simulink model "uGrid_1PH_hd_ATD3"  (R2018a)
settings: Solver=ode45  StartTime=0.0  StopTime=1.5  FixedStep=1e-6  MaxStep=1e-4  RelTol=1e-3
PreLoadFcn:
  | SimulinkInit
InitFcn:
  | SimulinkInit
StopFcn:
  | EndingScript
values from neighbouring files (symbols this model uses):
  Ad = sysd.A    [SimulinkInit.m]
  b = 4.91    [SimulinkInit.m]    (also in parametros_BIO.m)
  Bd = sysd.B    [SimulinkInit.m]
  C = 1    [SimulinkInit.m]    (also in parametros_BIO.m)
  C1 = Cd(2,:)    [SimulinkInit.m]
  C10 = Cd(1,:)    [SimulinkInit.m]
  C11 = Cd(2,:)    [SimulinkInit.m]
  C12 = Cd(3,:)    [SimulinkInit.m]
  C2 = Cd(3,:)    [SimulinkInit.m]
  C3 = Cd(4,:)    [SimulinkInit.m]
  C4 = Cd(1,:)    [SimulinkInit.m]
  C5 = Cd(3,:)    [SimulinkInit.m]
  C6 = Cd(4,:)    [SimulinkInit.m]
  C7 = Cd(1,:)    [SimulinkInit.m]
  C8 = Cd(2,:)    [SimulinkInit.m]
  C9 = Cd(4,:)    [SimulinkInit.m]
  Cd = sysd.C    [SimulinkInit.m]
  K = 25    [SimulinkInit.m]    (also in parametros_BIO.m; uio_linear.m = K1+E*H)
  K1 = 9.66    [SimulinkInit.m]    (also in parametros_BIO.m; uio_linear.m = K1')
  K11 = 0.8    [SimulinkInit.m]    (also in parametros_BIO.m)
  K2 = 6.97    [SimulinkInit.m]    (also in parametros_BIO.m)
  K22 = 0.2    [SimulinkInit.m]    (also in parametros_BIO.m)
  K3 = 31.8    [SimulinkInit.m]    (also in parametros_BIO.m)
  K33 = 0.23    [SimulinkInit.m]    (also in parametros_BIO.m)
  K4 = 15.1    [SimulinkInit.m]    (also in parametros_BIO.m)
  Kd = 0.02    [SimulinkInit.m]    (also in parametros_BIO.m)
  Kdc = 0.02    [SimulinkInit.m]    (also in parametros_BIO.m)
  Kf = 1    [SimulinkInit.m]    (also in parametros_BIO.m)
  Kh = 1.2    [SimulinkInit.m]    (also in parametros_BIO.m)
  Ks = 21.5    [SimulinkInit.m]    (also in parametros_BIO.m)
  Ksc = 3    [SimulinkInit.m]    (also in parametros_BIO.m)
  Kv = 1    [SimulinkInit.m]    (also in parametros_BIO.m)
  Sbin = 13.8    [SimulinkInit.m]    (also in parametros_BIO.m)
  Svin = 2.91    [SimulinkInit.m]    (also in parametros_BIO.m)
  T1 = 0.4    [parametros_BIO.m]
  T1s = 0.4    [SimulinkInit.m]
  T2 = 1    [parametros_BIO.m]
  T2s = 1    [SimulinkInit.m]
  T3 = 15    [parametros_BIO.m]
  T3s = 15    [SimulinkInit.m]
  T4 = 2.5    [parametros_BIO.m]
  T4s = 2.5    [SimulinkInit.m]
  T5 = 3.3    [parametros_BIO.m]
  T5s = 3.3    [SimulinkInit.m]
  Tao1 = 0.5    [SimulinkInit.m]
  Tcd = 0.2    [SimulinkInit.m]    (also in parametros_BIO.m)
  Tcr = 0.01    [SimulinkInit.m]    (also in parametros_BIO.m)
  Tf = 0.04    [SimulinkInit.m]    (also in parametros_BIO.m)
  tm = 1e-4    (= 0.0001)    [SimulinkInit.m]
  Tr = 950    [SimulinkInit.m]    (also in parametros_BIO.m)
  Tt = 450    [SimulinkInit.m]    (also in parametros_BIO.m)
  Ttd = 0.04    [SimulinkInit.m]    (also in parametros_BIO.m)
  Tv = 0.05    [SimulinkInit.m]    (also in parametros_BIO.m)
  V = 20    [SimulinkInit.m]    (also in parametros_BIO.m)
  wref = 70000    [SimulinkInit.m]    (also in parametros_BIO.m)
  X_acid = 1.2    [SimulinkInit.m]    (also in parametros_BIO.m)
  X_meth = 0.35    [SimulinkInit.m]    (also in parametros_BIO.m)
  Z = 3    [SimulinkInit.m]    (also in parametros_BIO.m)
undefined symbols (not defined in the file or in its folder): F1, F10, F11, F12, F2, F3, F4, F5, F6, F7, F8, F9, G, GF, H1, H10, H11, H12, H2, H3, H4, H5, H6, H7, H8, H9, Ion, K10U, K11U, K12U, K1U, K2U, K3U, K4U, K5U, K6U, K7U, K8U, K9U, Lithium, ss1, ss2, T10, T11, T12, T6, T7, T8, T9
libraries: powerlib x58, dsparch4 x16, truetime x12, powerlib_meascontrol x6, dspstat3 x2, simulink x1, electricdrivelib x1
(part 2 of 3)

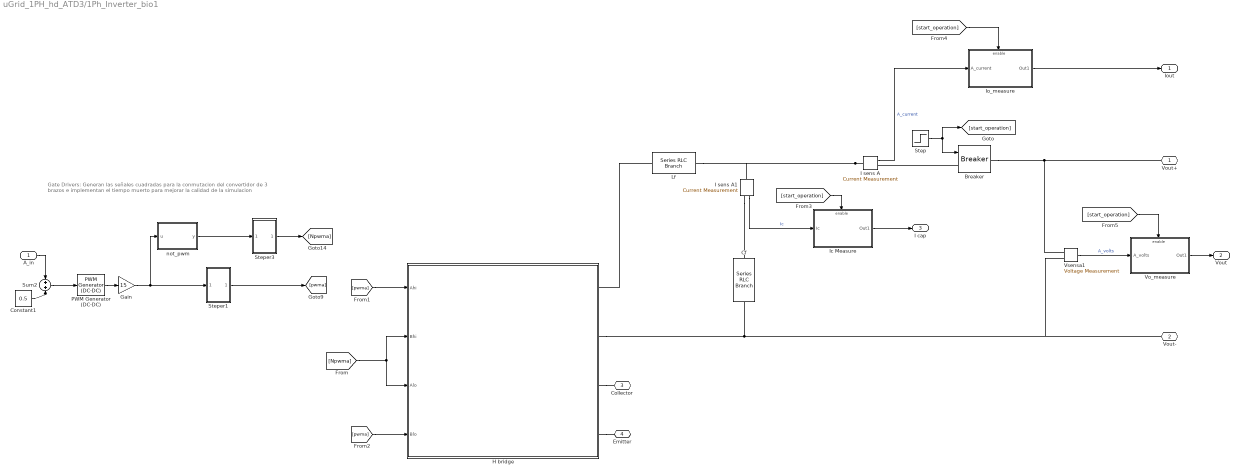
== system uGrid_1PH_hd_ATD3/1Ph_Inverter_bio1 ==
  note: Gate Drivers: Generan las señales cuadradas para
      | la conmutacion del convertidor de 3 brazos e implementan el
      | tiempo muerto para mejorar la calidad de la simulacion
  A_in : Inport
  Breaker : powerlib/Elements/Breaker  InitialState=0  SwitchingTimes="[1/60  5/60]"  External=on  BreakerResistance=0.01  SnubberResistance=1e6  SnubberCapacitance=inf  Measurements=None  MoreParameters=on  NoBreakLoop=off
      settings: SourceProductName=Simscape Power Systems
  Cf : powerlib/Elements/Series RLC Branch  LConnTagsString=__new0  RConnTagsString=__new0  BranchType=C  Resistance=1  Inductance=1e-3  SetiL0=off  InitialCurrent=0  Capacitance=610e-6  Setx0=off  InitialVoltage=0  Measurements=None
  Constant1 : Constant  Value=0.5
  Gain : Gain  Gain=15
  H bridge : Subsystem
      mask Display:
      | port_label('input', 1, '\fontsize{12} Ahi', 'texmode', 'on')
      | port_label('input', 2, '\fontsize{12} Alo', 'texmode', 'on')
      | port_label('input', 3, '\fontsize{12} Bhi', 'texmode', 'on')
      | port_label('input', 4, '\fontsize{12} Blo', 'texmode', 'on')
      | 
      | 
      | port_label('rconn', 1, '\fontsize{12} V_{out} +', 'texmode', 'on')
      | port_label('rconn', 2, '\fontsize{12} V_{out} -', 'texmode', 'on')
      | 
      | port_label('rconn', 3, '\fontsize{12} Collector', 'texmode', 'on')
      | port_label('rconn', 4, '\fontsize{12} Emitter', 'texmode', 'on')
      | 
      | lvx = [.1 .1];
      | lvy = [.1 .2];
      | lhx = [.1 .2];
      | lhy = [.1 .1];
      | 
      | 
      | % se dibujan los interruptores de la izquierda
      | plot(lvx+.07, lvy*.8+.028+.1)
      | plot(lvx+.1, lvy+.1)
      | plot(lhx*.5+.15, lhy+.1)
      | plot(lhx*.5+.15, lhy+.2)
      | plot(lhx*.5+.07, lhy+.15)
      | 
      | d=0.5;
      | 
      | plot(lvx+.07, lvy*.8+.028+.1+d)
      | plot(lvx+.1, lvy+.1+d)
      | plot(lhx*.5+.15, lhy+.1+d)
      | plot(lhx*.5+.15, lhy+.2+d)
      | plot(lhx*.5+.07, lhy+.15+d)
      | 
      | 
      | % se dibujan los interruptores del medio
      | h=.3;
      | 
      | %plot(lvx+.07+h, lvy*.8+.028+.1)
      | %plot(lvx+.1+h, lvy+.1)
      | %plot(lhx*.5+.15+h, lhy+.1)
      | %plot(lhx*.5+.15+h, lhy+.2)
      | %plot(lhx*.5+.07+h, lhy+.15)
      | 
      | %plot(lvx+.07+h, lvy*.8+.028+.1+d)
      | %plot(lvx+.1+h, lvy+.1+d)
      | %plot(lhx*.5+.15+h, lhy+.1+d)
      | %plot(lhx*.5+.15+h, lhy+.2+d)
      | %plot(lhx*.5+.07+h, lhy+.15+d)
      | 
      | % se dibujan los interruptores de la derecha
      | h=.6
      | 
      | plot(lvx+.07+h, lvy*.8+.028+.1)
      | plot(lvx+.1+h, lvy+.1)
      | plot(lhx*.5+.15+h, lhy+.1)
      | plot(lhx*.5+.15+h, lhy+.2)
      | plot(lhx*.5+.07+h, lhy+.15)
      | 
      | plot(lvx+.07+h, lvy*.8+.028+.1+d)
      | plot(lvx+.1+h, lvy+.1+d)
      | plot(lhx*.5+.15+h, lhy+.1+d)
      | plot(lhx*.5+.15+h, lhy+.2+d)
      | plot(lhx*.5+.07+h, lhy+.15+d)
      | 
      | 
      | % se conectan los interruptores.
      | plot(lvx+.15, lvy*4-.1)
      | %plot(lvx+.15+.3, lvy*4-.1)
      | plot(lvx+.15+.6, lvy*4-.1)
      | 
      | 
      | plot(lvx+.15, lvy+.7)
      | %plot(lvx+.15+.3, lvy+.7)
      | plot(lvx+.15+.6, lvy+.7)
      | 
      | plot(lvx+.15, lvy)
      | %plot(lvx+.15+.3, lvy)
      | plot(lvx+.15+.6, lvy)
      | 
      | plot(lhx*6-.35, lhy)
      | plot(lhx*6-.35, lhy+.8)
      | 
      | % raul esteban alzate 313 515 86 11
  I sens A : powerlib/Measurements/Current Measurement  PhasorSimulation=off  OutputType=Complex  PSBequivalent=0
  I sens A1 : powerlib/Measurements/Current Measurement  PhasorSimulation=off  OutputType=Complex  PSBequivalent=0
  Ic Measure : Subsystem
  Io_measure : Subsystem
  Lf : powerlib/Elements/Series RLC Branch  LConnTagsString=__new0  RConnTagsString=__new0  BranchType=RL  Resistance=1e-3  Inductance=5e-3  SetiL0=off  InitialCurrent=0  Capacitance=1e-6  Setx0=off  InitialVoltage=0  Measurements=None
  PWM Generator (DC-DC) : powerlib_meascontrol/Pulse & Signal Generators/PWM Generator (DC-DC)  Fsw=f_sw  Ts=samp_f
  Step : Step  Time=st_time  SampleTime=0
  Steper1 : Subsystem
  Steper3 : Subsystem
  Sum2 : Sum
  Vo_measure : Subsystem
  Vsensa1 : powerlib/Measurements/Voltage Measurement  PhasorSimulation=off  OutputType=Complex  PSBequivalent=0
  not_pwm : MATLAB Function  TreatAsAtomicUnit=on
  Vout+ : PMIOPort  Side=Right
  Vout- : PMIOPort  Port=2  Side=Right
  Collector : PMIOPort  Port=3  Side=Left
  Emitter : PMIOPort  Port=4  Side=Left
  Iout : Outport
  Vout : Outport  Port=2
  I cap : Outport  Port=3
  wires:
  not_pwm/1(y) -> Steper3/1(In1)
  Sum2/1 -> PWM Generator (DC-DC)/1
  PWM Generator (DC-DC)/1 -> Gain/1
  Constant1/1 -> Sum2/2
  A_in/1 -> Sum2/1
  Steper1/1(Out1) -> [pwma]
  Steper3/1(Out1) -> [Npwma]
  Gain/1 -> Steper1/1(In1), not_pwm/1(u)
  [pwma] -> H bridge/1(Ahi)
  [Npwma] -> H bridge/2(Bhi), H bridge/3(Alo)
  [pwma] -> H bridge/4(Blo)
  Step/1 -> [start_operation], Breaker/1
  I sens A1/1 -> Ic Measure/1(Ic)  "Ic"
  Ic Measure/1(Out1) -> I cap/1
  [start_operation] -> Ic Measure/Enable
  Vsensa1/1 -> Vo_measure/1(A_volts)  "A_volts"
  Vo_measure/1(Out1) -> Vout/1
  I sens A/1 -> Io_measure/1(A_current)  "A_current"
  Io_measure/1(Out1) -> Iout/1
  [start_operation] -> Io_measure/Enable
  [start_operation] -> Vo_measure/Enable
  connections:
  H bridge/RConn3 -- Collector/RConn1
  H bridge/RConn4 -- Emitter/RConn1
  Lf/LConn1 -- H bridge/RConn1
  H bridge/RConn2 -- Vout-/RConn1 -- Vsensa1/LConn2 -- Cf/RConn1
  Breaker/LConn1 -- I sens A/RConn1
  Breaker/RConn1 -- Vsensa1/LConn1 -- Vout+/RConn1
  I sens A/LConn1 -- Lf/RConn1 -- I sens A1/LConn1
  I sens A1/RConn1 -- Cf/LConn1

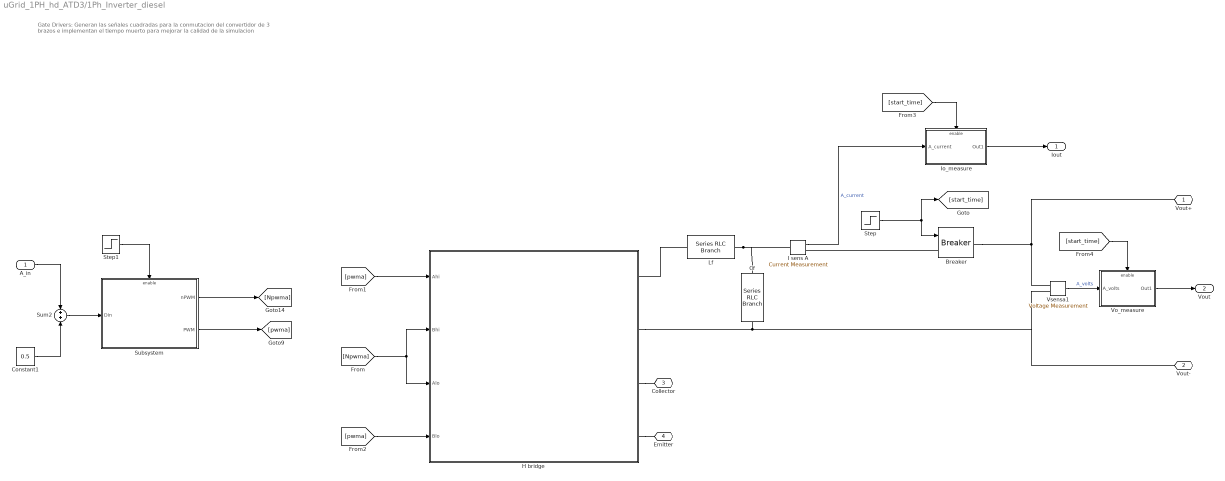
== system uGrid_1PH_hd_ATD3/1Ph_Inverter_diesel ==
  note: Gate Drivers: Generan las señales cuadradas para
      | la conmutacion del convertidor de 3 brazos e implementan el
      | tiempo muerto para mejorar la calidad de la simulacion
  A_in : Inport
  Breaker : powerlib/Elements/Breaker  InitialState=0  SwitchingTimes="[1/60  5/60]"  External=on  BreakerResistance=0.01  SnubberResistance=1e6  SnubberCapacitance=inf  Measurements=None  MoreParameters=on  NoBreakLoop=off
      settings: SourceProductName=Simscape Power Systems
  Cf : powerlib/Elements/Series RLC Branch  LConnTagsString=__new0  RConnTagsString=__new0  BranchType=C  Resistance=1  Inductance=1e-3  SetiL0=off  InitialCurrent=0  Capacitance=22e-6  Setx0=off  InitialVoltage=0  Measurements=None
  Constant1 : Constant  Value=0.5
  H bridge : Subsystem
      mask Display:
      | port_label('input', 1, '\fontsize{12} Ahi', 'texmode', 'on')
      | port_label('input', 2, '\fontsize{12} Alo', 'texmode', 'on')
      | port_label('input', 3, '\fontsize{12} Bhi', 'texmode', 'on')
      | port_label('input', 4, '\fontsize{12} Blo', 'texmode', 'on')
      | 
      | 
      | port_label('rconn', 1, '\fontsize{12} V_{out} +', 'texmode', 'on')
      | port_label('rconn', 2, '\fontsize{12} V_{out} -', 'texmode', 'on')
      | 
      | port_label('rconn', 3, '\fontsize{12} Collector', 'texmode', 'on')
      | port_label('rconn', 4, '\fontsize{12} Emitter', 'texmode', 'on')
      | 
      | lvx = [.1 .1];
      | lvy = [.1 .2];
      | lhx = [.1 .2];
      | lhy = [.1 .1];
      | 
      | 
      | % se dibujan los interruptores de la izquierda
      | plot(lvx+.07, lvy*.8+.028+.1)
      | plot(lvx+.1, lvy+.1)
      | plot(lhx*.5+.15, lhy+.1)
      | plot(lhx*.5+.15, lhy+.2)
      | plot(lhx*.5+.07, lhy+.15)
      | 
      | d=0.5;
      | 
      | plot(lvx+.07, lvy*.8+.028+.1+d)
      | plot(lvx+.1, lvy+.1+d)
      | plot(lhx*.5+.15, lhy+.1+d)
      | plot(lhx*.5+.15, lhy+.2+d)
      | plot(lhx*.5+.07, lhy+.15+d)
      | 
      | 
      | % se dibujan los interruptores del medio
      | h=.3;
      | 
      | %plot(lvx+.07+h, lvy*.8+.028+.1)
      | %plot(lvx+.1+h, lvy+.1)
      | %plot(lhx*.5+.15+h, lhy+.1)
      | %plot(lhx*.5+.15+h, lhy+.2)
      | %plot(lhx*.5+.07+h, lhy+.15)
      | 
      | %plot(lvx+.07+h, lvy*.8+.028+.1+d)
      | %plot(lvx+.1+h, lvy+.1+d)
      | %plot(lhx*.5+.15+h, lhy+.1+d)
      | %plot(lhx*.5+.15+h, lhy+.2+d)
      | %plot(lhx*.5+.07+h, lhy+.15+d)
      | 
      | % se dibujan los interruptores de la derecha
      | h=.6
      | 
      | plot(lvx+.07+h, lvy*.8+.028+.1)
      | plot(lvx+.1+h, lvy+.1)
      | plot(lhx*.5+.15+h, lhy+.1)
      | plot(lhx*.5+.15+h, lhy+.2)
      | plot(lhx*.5+.07+h, lhy+.15)
      | 
      | plot(lvx+.07+h, lvy*.8+.028+.1+d)
      | plot(lvx+.1+h, lvy+.1+d)
      | plot(lhx*.5+.15+h, lhy+.1+d)
      | plot(lhx*.5+.15+h, lhy+.2+d)
      | plot(lhx*.5+.07+h, lhy+.15+d)
      | 
      | 
      | % se conectan los interruptores.
      | plot(lvx+.15, lvy*4-.1)
      | %plot(lvx+.15+.3, lvy*4-.1)
      | plot(lvx+.15+.6, lvy*4-.1)
      | 
      | 
      | plot(lvx+.15, lvy+.7)
      | %plot(lvx+.15+.3, lvy+.7)
      | plot(lvx+.15+.6, lvy+.7)
      | 
      | plot(lvx+.15, lvy)
      | %plot(lvx+.15+.3, lvy)
      | plot(lvx+.15+.6, lvy)
      | 
      | plot(lhx*6-.35, lhy)
      | plot(lhx*6-.35, lhy+.8)
      | 
      | % raul esteban alzate 313 515 86 11
  I sens A : powerlib/Measurements/Current Measurement  PhasorSimulation=off  OutputType=Complex  PSBequivalent=0
  Io_measure : Subsystem
  Lf : powerlib/Elements/Series RLC Branch  LConnTagsString=__new0  RConnTagsString=__new0  BranchType=RL  Resistance=.1  Inductance=30e-3  SetiL0=off  InitialCurrent=0  Capacitance=1e-6  Setx0=off  InitialVoltage=0  Measurements=None
  Step : Step  Time=st_time  SampleTime=0
  Step1 : Step  Time=st_time  SampleTime=0
  Subsystem : Subsystem
  Sum2 : Sum
  Vo_measure : Subsystem
  Vsensa1 : powerlib/Measurements/Voltage Measurement  PhasorSimulation=off  OutputType=Complex  PSBequivalent=0
  Vout+ : PMIOPort  Side=Right
  Vout- : PMIOPort  Port=2  Side=Right
  Collector : PMIOPort  Port=3  Side=Left
  Emitter : PMIOPort  Port=4  Side=Left
  Iout : Outport
  Vout : Outport  Port=2
  wires:
  [pwma] -> H bridge/4(Blo)
  [Npwma] -> H bridge/3(Alo), H bridge/2(Bhi)
  [pwma] -> H bridge/1(Ahi)
  A_in/1 -> Sum2/1
  Constant1/1 -> Sum2/2
  Step/1 -> [start_time], Breaker/1
  Sum2/1 -> Subsystem/1(Din)
  Subsystem/1(nPWM) -> [Npwma]
  Subsystem/2(PWM) -> [pwma]
  Step1/1 -> Subsystem/Enable
  Vsensa1/1 -> Vo_measure/1(A_volts)  "A_volts"
  Vo_measure/1(Out1) -> Vout/1
  I sens A/1 -> Io_measure/1(A_current)  "A_current"
  Io_measure/1(Out1) -> Iout/1
  [start_time] -> Io_measure/Enable
  [start_time] -> Vo_measure/Enable
  connections:
  Cf/RConn1 -- Vsensa1/LConn2 -- Vout-/RConn1 -- H bridge/RConn2
  Lf/LConn1 -- H bridge/RConn1
  H bridge/RConn4 -- Emitter/RConn1
  H bridge/RConn3 -- Collector/RConn1
  Breaker/LConn1 -- I sens A/RConn1
  Breaker/RConn1 -- Vsensa1/LConn1 -- Vout+/RConn1
  Lf/RConn1 -- I sens A/LConn1 -- Cf/LConn1

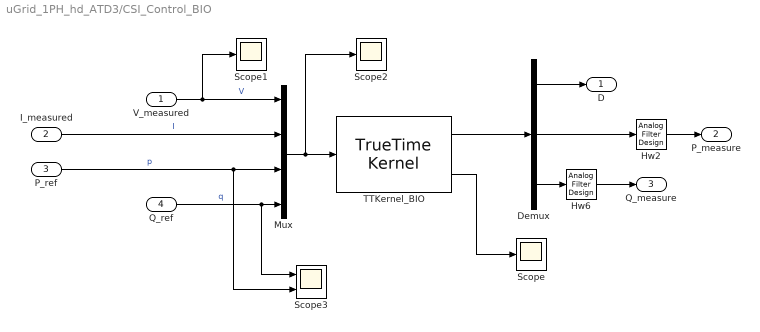
== system uGrid_1PH_hd_ATD3/CSI_Control_BIO ==
  V_measured : Inport
  I_measured : Inport  Port=2
  P_ref : Inport  Port=3
  Q_ref : Inport  Port=4
  Demux : Demux  Outputs=3
  Hw2 : dsparch4/Analog Filter Design  method=Bessel  filttype=Lowpass  N=4  Wlo=30*2*pi  Whi=80  Rp=2  Rs=80
  Hw6 : dsparch4/Analog Filter Design  method=Bessel  filttype=Lowpass  N=4  Wlo=30*2*pi  Whi=80  Rp=2  Rs=80
  Mux : Mux
  Scope : Scope
  Scope1 : Scope
  Scope2 : Scope
  Scope3 : Scope  NumInputPorts=2
  TTKernel_BIO : truetime/TrueTime Kernel  sfun=BIO_init  args=1  ninputsoutputs=[4 3]  ntriggers=0  trigtype=falling  nwnodenbr=[]  clockoffsetdrift=[0 0]  schedoutput=on  battery=off  poweroutput=off
  D : Outport
  P_measure : Outport  Port=2
  Q_measure : Outport  Port=3
  wires:
  TTKernel_BIO/1 -> Demux/1
  Demux/3 -> Hw6/1
  Demux/2 -> Hw2/1
  Demux/1 -> D/1
  TTKernel_BIO/2 -> Scope/1
  Mux/1 -> Scope2/1, TTKernel_BIO/1
  V_measured/1 -> Scope1/1, Mux/1  "V"
  I_measured/1 -> Mux/2  "I"
  P_ref/1 -> Scope3/2, Mux/3  "p"
  Q_ref/1 -> Scope3/1, Mux/4  "q"
  Hw6/1 -> Q_measure/1
  Hw2/1 -> P_measure/1

== system uGrid_1PH_hd_ATD3/CSI_Control_DIESEL ==
  V_measured : Inport
  I_measured : Inport  Port=2
  P_ref : Inport  Port=3
  Q_ref : Inport  Port=4
  Demux : Demux  Outputs=3
  Hw1 : dsparch4/Analog Filter Design  method=Bessel  filttype=Lowpass  N=4  Wlo=30*2*pi  Whi=80  Rp=2  Rs=80
  Hw3 : dsparch4/Analog Filter Design  method=Bessel  filttype=Lowpass  N=4  Wlo=30*2*pi  Whi=80  Rp=2  Rs=80
  Mux : Mux
  TTKernel_DIESEL : truetime/TrueTime Kernel  sfun=DIESEL_init  args=[]  ninputsoutputs=[4 3]  ntriggers=0  trigtype=falling  nwnodenbr=[]  clockoffsetdrift=[0 0]  schedoutput=on  battery=off  poweroutput=off
  D : Outport
  P_measure : Outport  Port=2
  Q_measure : Outport  Port=3
  wires:
  Mux/1 -> TTKernel_DIESEL/1
  Demux/3 -> Hw3/1
  Demux/2 -> Hw1/1
  TTKernel_DIESEL/1 -> Demux/1
  Demux/1 -> D/1
  Hw1/1 -> P_measure/1
  Hw3/1 -> Q_measure/1
  P_ref/1 -> Mux/3
  Q_ref/1 -> Mux/4
  I_measured/1 -> Mux/2
  V_measured/1 -> Mux/1

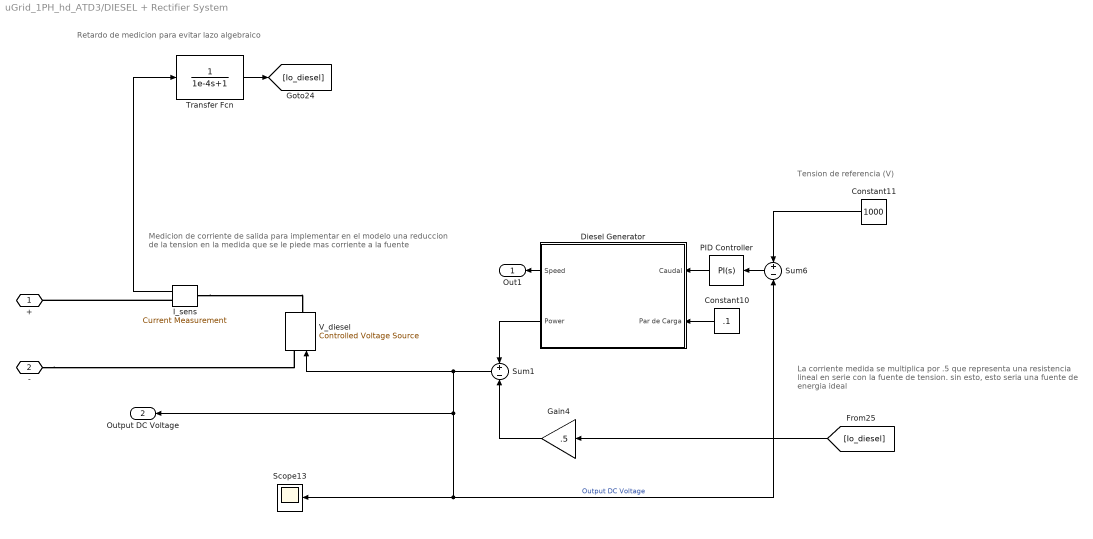
== system uGrid_1PH_hd_ATD3/DIESEL + Rectifier System ==
  note: Tension de referencia (V)
  note: La corriente medida se multiplica por .5 que
      | representa una resistencia lineal en serie con
      | la fuente de tension. sin esto, esto seria una
      | fuente de energia ideal
  note: Medicion de corriente de salida para implementar
      | en el modelo una reduccion de la tension en la
      | medida que se le piede mas corriente a la fuente
  note: Retardo de medicion para evitar lazo algebraico
  Constant10 : Constant  Value=.1
  Constant11 : Constant  Value=1000
  Diesel Generator : Subsystem
  Gain4 : Gain  Gain=.5
  I_sens : powerlib/Measurements/Current Measurement  PhasorSimulation=off  OutputType=Complex  PSBequivalent=0
  PID Controller : simulink/Continuous/PID Controller  Controller=PI  TimeDomain=Continuous-time  SampleTime=-1  IntegratorMethod=Forward Euler  FilterMethod=Forward Euler  Form=Parallel  UseFilter=on  ControllerParametersSource=internal  P=0.00325909628031494  I=0.000326732379168699  D=0.00124823483730586  N=0.606508283225141  InitialConditionSource=internal  InitialConditionForIntegrator=0.248  InitialConditionForFilter=0.24  ExternalReset=none  LimitOutput=off  UpperSaturationLimit=inf  LowerSaturationLimit=-inf  LinearizeAsGain=on  AntiWindupMode=none  Kb=1  TrackingMode=off  Kt=1  PParamMin=[]  PParamMax=[]  IParamMin=[]  IParamMax=[]  DParamMin=[]  DParamMax=[]  NParamMin=[]  NParamMax=[]  KbParamMin=[]  KbParamMax=[]  KtParamMin=[]  KtParamMax=[]  POutMin=[]  POutMax=[]  IOutMin=[]  IOutMax=[]  DOutMin=[]  DOutMax=[]  NOutMin=[]  NOutMax=[]  KbOutMin=[]  KbOutMax=[]  KtOutMin=[]  KtOutMax=[]  IntegratorOutMin=[]  IntegratorOutMax=[]  FilterOutMin=[]  FilterOutMax=[]  SumOutMin=[]  SumOutMax=[]  SumI1OutMin=[]  SumI1OutMax=[]  SumI2OutMin=[]  SumI2OutMax=[]  SumI3OutMin=[]  SumI3OutMax=[]  SumDOutMin=[]  SumDOutMax=[]  SaturationOutMin=[]  SaturationOutMax=[]  IntegratorContinuousStateAttributes=''  IntegratorStateMustResolveToSignalObject=off  IntegratorRTWStateStorageClass=Auto  FilterContinuousStateAttributes=''  FilterStateMustResolveToSignalObject=off  FilterRTWStateStorageClass=Auto  DifferentiatorICPrevScaledInput=0  DifferentiatorOutMin=[]  DifferentiatorOutMax=[]  InitialConditionSetting=State (most efficient)  FilterDiffOutCoefMin=[]  FilterDiffOutCoefMax=[]  SumDenOutMin=[]  SumDenOutMax=[]  SumNumOutMin=[]  SumNumOutMax=[]  ReciprocalOutMin=[]  ReciprocalOutMax=[]  DivideOutMin=[]  DivideOutMax=[]  TunerSelectOption=Transfer Function Based (PID Tuner App)
  Scope13 : Scope
  Sum1 : Sum  Inputs=+-
  Sum6 : Sum  Inputs=+-
  Transfer Fcn : TransferFcn  Denominator=[1e-4 1]
  V_diesel : powerlib/Electrical Sources/Controlled Voltage Source  Initialize=on  Source_Type=AC  Amplitude=0  Phase=0  Frequency=0  Measurements=None
  + : PMIOPort  Side=Left
  - : PMIOPort  Port=2  Side=Left
  Out1 : Outport
  Output DC Voltage : Outport  Port=2
  wires:
  Sum1/1 -> Output DC Voltage/1, Sum6/2, Scope13/1, V_diesel/1  "Output DC Voltage"
  Transfer Fcn/1 -> [Io_diesel]
  I_sens/1 -> Transfer Fcn/1
  Diesel Generator/2(Power) -> Sum1/1
  Sum6/1 -> PID Controller/1
  Diesel Generator/1(Speed) -> Out1/1
  Gain4/1 -> Sum1/2
  Constant10/1 -> Diesel Generator/2(Par de Carga)
  Constant11/1 -> Sum6/1
  [Io_diesel] -> Gain4/1
  PID Controller/1 -> Diesel Generator/1(Caudal)
  connections:
  -/RConn1 -- V_diesel/LConn1
  I_sens/LConn1 -- V_diesel/RConn1
  I_sens/RConn1 -- +/RConn1

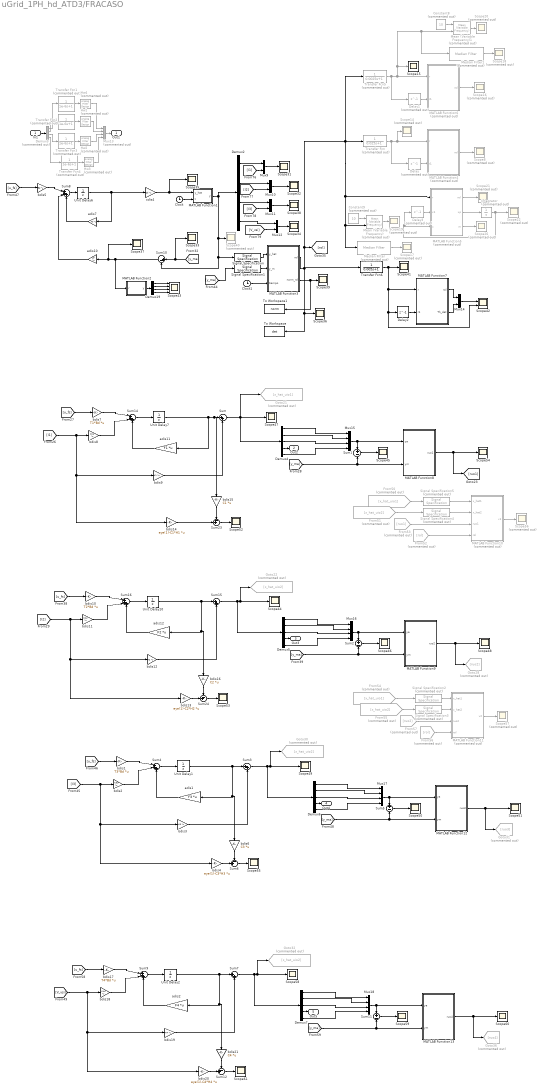
== system uGrid_1PH_hd_ATD3/FRACASO ==
  In1 : Inport
  Clock : Clock
  Clock1 : Clock
  Constant8 : Constant  Commented=on  Value=10
  Constant9 : Constant  Commented=on  Value=10
  Delay : Delay  Commented=on  DelayLength=1
  Delay1 : Delay  Commented=on  DelayLength=1
  Delay2 : Delay  DelayLength=1
  Delay3 : Delay  Commented=on  DelayLength=1
  Demux19 : Demux
  Demux2 : Demux
  Demux3 : Demux  Commented=on
  Demux{4..7} (4 alike) : Demux  Outputs=5
  From50 : From  Commented=on  GotoTag=x_hat_uio1
  From51 : From  Commented=on  GotoTag=x_hat_uio2
  From52 : From  Commented=on  GotoTag=rol
  From53 : From  Commented=on  GotoTag=ruo1
  From54 : From  Commented=on  GotoTag=x_hat_uio1
  From55 : From  Commented=on  GotoTag=x_hat_uio2
  From56 : From  Commented=on  GotoTag=rol
  From57 : From  Commented=on  GotoTag=ruo2
  Goto21 : Goto  Commented=on  GotoTag=x_hat_uio1
  Goto22 : Goto  Commented=on  GotoTag=x_hat_uio2
  Goto28 : Goto  Commented=on  GotoTag=ruo2
  Goto30 : Goto  Commented=on  GotoTag=x_hat_uio2
  Goto31 : Goto  Commented=on  GotoTag=ruo3
  Goto32 : Goto  Commented=on  GotoTag=x_hat_uio2
  Goto36 : Goto  Commented=on  GotoTag=ruo4
  Hw{1..4} (4 alike) : dsparch4/Analog Filter Design  Commented=on  method=Bessel  filttype=Lowpass  N=2  Wlo=7000*2*pi  Whi=80  Rp=2  Rs=80
  Integrator : Integrator  Commented=on
  MATLAB Function1 : MATLAB Function  TreatAsAtomicUnit=on
  MATLAB Function10 : MATLAB Function  Commented=on  TreatAsAtomicUnit=on
  MATLAB Function11 : MATLAB Function  Commented=on  TreatAsAtomicUnit=on
  MATLAB Function12 : MATLAB Function  TreatAsAtomicUnit=on
  MATLAB Function13 : MATLAB Function  TreatAsAtomicUnit=on
  MATLAB Function2 : MATLAB Function  TreatAsAtomicUnit=on
  MATLAB Function3 : MATLAB Function  TreatAsAtomicUnit=on
  MATLAB Function4 : MATLAB Function  Commented=on  TreatAsAtomicUnit=on
  MATLAB Function5 : MATLAB Function  Commented=on  TreatAsAtomicUnit=on
  MATLAB Function6 : MATLAB Function  Commented=on  TreatAsAtomicUnit=on
  MATLAB Function7 : MATLAB Function  TreatAsAtomicUnit=on
  MATLAB Function8 : MATLAB Function  TreatAsAtomicUnit=on
  MATLAB Function9 : MATLAB Function  TreatAsAtomicUnit=on
  Mean (Variable Frequency) : powerlib_meascontrol/Measurements/Mean (Variable Frequency)  Commented=on  Finit=60  Fmin=45  Vinit=0  Ts=0
      settings: SourceProductName=Simscape Power Systems  SourceProductBaseCode=PS
  Mean (Variable Frequency)1 : powerlib_meascontrol/Measurements/Mean (Variable Frequency)  Commented=on  Finit=60  Fmin=45  Vinit=0  Ts=0
      settings: SourceProductName=Simscape Power Systems  SourceProductBaseCode=PS
  Median Filter : dspstat3/Median Filter  Commented=on  WindowLength=100  SimulateUsing=Interpreted execution
      settings: SourceProductName=DSP System Toolbox  SourceProductBaseCode=DS
  Median Filter1 : dspstat3/Median Filter  Commented=on  WindowLength=100  SimulateUsing=Interpreted execution
      settings: SourceProductName=DSP System Toolbox  SourceProductBaseCode=DS
  Mux{9..12,14} (5 alike) : Mux  Inputs=2
  Mux13 : Mux  Commented=on
  Mux{15..18} (4 alike) : Mux
  Scope{8,14,16..22,26,40,56..57} (13 alike) : Scope  Commented=on
  Scope{15,31..39,41,44..55,58..61} (27 alike) : Scope
  Scope42 : Scope  NumInputPorts=2
  Scope43 : Scope  NumInputPorts=4
  Signal Specification : SignalSpecification  Dimensions=4
  Signal Specification1 : SignalSpecification  Dimensions=4
  Signal Specification{2..5} (4 alike) : SignalSpecification  Commented=on  Dimensions=3
  Sum{,3,7,15} (4 alike) : Sum  Inputs=|++
  Sum{1..2,5,11} (4 alike) : Sum  Inputs=+-
  Sum10 : Sum  Inputs=|+-
  Sum{6,12,23..24} (4 alike) : Sum  Inputs=-+|
  Sum{4,8..9,14,16} (5 alike) : Sum  Inputs=|+++  SampleTime=tm
  To Workspace : ToWorkspace  VariableName=det  SampleTime=1e-4
  To Workspace1 : ToWorkspace  VariableName=norm  SampleTime=1e-4
  Transfer Fcn : TransferFcn  Commented=on  Denominator=[0.025 1]
  Transfer Fcn{1..4} (4 alike) : TransferFcn  Commented=on  Denominator=[1e-6 1]
  Transfer Fcn5 : TransferFcn  Commented=on  Denominator=[0.0025 1]
  Transfer Fcn6 : TransferFcn  Denominator=[0.005 1]
  Unit Delay{1..2,6..7,10} (5 alike) : UnitDelay  SampleTime=tm
  adis1 : Gain  Gain=F3  Multiplication=Matrix(K*u) (u vector)  SampleTime=tm
  adis10 : Gain  Gain=Ld'  Multiplication=Matrix(K*u) (u vector)  SampleTime=tm
  adis11 : Gain  Gain=F1  Multiplication=Matrix(K*u) (u vector)  SampleTime=tm
  adis12 : Gain  Gain=F2  Multiplication=Matrix(K*u) (u vector)  SampleTime=tm
  adis2 : Gain  Gain=F4  Multiplication=Matrix(K*u) (u vector)  SampleTime=tm
  adis7 : Gain  Gain=Ad  Multiplication=Matrix(K*u) (u vector)  SampleTime=tm
  bdis1 : Gain  Gain=T3*Bd  Multiplication=Matrix(K*u) (u vector)  SampleTime=tm
  bdis10 : Gain  Gain=T2*Bd  Multiplication=Matrix(K*u) (u vector)  SampleTime=tm
  bdis11 : Gain  Gain=K2U  Multiplication=Matrix(K*u) (u vector)  SampleTime=tm
  bdis12 : Gain  Gain=H2  Multiplication=Matrix(K*u) (u vector)  SampleTime=tm
  bdis13 : Gain  Gain=eye(1)-C2*H2  Multiplication=Matrix(K*u) (u vector)  SampleTime=tm
  bdis14 : Gain  Gain=eye(1)-C1*H1  Multiplication=Matrix(K*u) (u vector)  SampleTime=tm
  bdis15 : Gain  Gain=C1  Multiplication=Matrix(K*u) (u vector)  SampleTime=tm
  bdis16 : Gain  Gain=C2  Multiplication=Matrix(K*u) (u vector)  SampleTime=tm
  bdis17 : Gain  Gain=T4*Bd  Multiplication=Matrix(K*u) (u vector)  SampleTime=tm
  bdis18 : Gain  Gain=K4U  Multiplication=Matrix(K*u) (u vector)  SampleTime=tm
  bdis19 : Gain  Gain=H4  Multiplication=Matrix(K*u) (u vector)  SampleTime=tm
  bdis2 : Gain  Gain=K3U  Multiplication=Matrix(K*u) (u vector)  SampleTime=tm
  bdis20 : Gain  Gain=eye(1)-C4*H4  Multiplication=Matrix(K*u) (u vector)  SampleTime=tm
  bdis21 : Gain  Gain=C4  Multiplication=Matrix(K*u) (u vector)  SampleTime=tm
  bdis3 : Gain  Gain=H3  Multiplication=Matrix(K*u) (u vector)  SampleTime=tm
  bdis4 : Gain  Gain=eye(1)-C3*H3  Multiplication=Matrix(K*u) (u vector)  SampleTime=tm
  bdis5 : Gain  Gain=Bd  Multiplication=Matrix(K*u) (u vector)  SampleTime=tm
  bdis6 : Gain  Gain=C3  Multiplication=Matrix(K*u) (u vector)  SampleTime=tm
  bdis7 : Gain  Gain=T1*Bd  Multiplication=Matrix(K*u) (u vector)  SampleTime=tm
  bdis8 : Gain  Gain=K1U  Multiplication=Matrix(K*u) (u vector)  SampleTime=tm
  bdis9 : Gain  Gain=H1  Multiplication=Matrix(K*u) (u vector)  SampleTime=tm
  cdis4 : Gain  Gain=Cd  Multiplication=Matrix(K*u) (u vector)  SampleTime=tm
  Out1 : Outport
  Out2 : Outport  Port=2
  Out3 : Outport  Port=3
  Out4 : Outport  Port=4
  Out5 : Outport  Port=5
  wires:
  Hw3/1 -> Mux13/4
  Demux19/1 -> Scope43/1
  Transfer Fcn5/1 -> Delay1/1, MATLAB Function6/1(r), Median Filter1/1, Mean (Variable Frequency)1/2, Scope15/1
  Signal Specification1/1 -> MATLAB Function3/2(y_m)
  [u_fs] -> bdis5/1
  Unit Delay6/1 -> cdis4/1, adis7/1
  Transfer Fcn6/1 -> Scope42/2, Delay2/1, MATLAB Function7/1(r), Scope41/1
  Demux3/4 -> Transfer Fcn4/1
  [y_ma] -> Scope33/1, Sum10/1
  Sum4/1 -> Unit Delay1/1
  bdis5/1 -> Sum8/1
  Demux2/4 -> Mux12/1
  adis10/1 -> Sum8/2
  Sum15/1 -> Demux5/1, Goto22/1, Scope44/1
  Integrator/1 -> Delay3/1, MATLAB Function5/3(x), Scope22/1
  [y_ma] -> Sum11/2, MATLAB Function13/2(ym)
  [y_ma] -> Sum1/2, MATLAB Function8/2(ym)
  Demux19/2 -> Scope43/2
  Demux2/1 -> Mux9/1
  Transfer Fcn3/1 -> Hw2/1
  Delay3/1 -> MATLAB Function5/2(x1)
  Demux6/3 -> Mux17/3
  Sum12/1 -> Scope61/1
  Transfer Fcn2/1 -> Hw1/1
  bdis3/1 -> Sum3/2
  [I1] -> Mux9/2
  Demux5/5 -> Mux16/4
  Median Filter/1 -> Scope17/1
  bdis8/1 -> Sum14/2
  Demux3/1 -> Transfer Fcn1/1
  Transfer Fcn/1 -> Delay/1, MATLAB Function4/1(r), Scope14/1
  MATLAB Function1/1(y) -> Demux2/1, Scope40/1, Sum10/2, Signal Specification/1
  Mux11/1 -> Scope38/1
  [u_fs] -> bdis17/1
  Mux12/1 -> Scope34/1
  MATLAB Function8/1(ruo1) -> [ruo1], Scope54/1
  [y_ma] -> Signal Specification1/1
  Mux9/1 -> Scope31/1
  Delay1/1 -> MATLAB Function6/2(r1)
  Sum10/1 -> MATLAB Function2/1(r), Scope37/1, adis10/1
  Constant8/1 -> Mean (Variable Frequency)1/1
  Demux2/2 -> Mux10/1
  MATLAB Function3/1(rol) -> MATLAB Function5/1(r), Median Filter/1, Mean (Variable Frequency)/2, Transfer Fcn5/1, Transfer Fcn/1, [rol], To Workspace/1, Scope36/1, Transfer Fcn6/1
  Demux19/3 -> Scope43/3
  Mux10/1 -> Scope32/1
  Demux2/3 -> Mux11/1
  Demux7/2 -> Mux18/2
  [y_ma] -> Sum2/2, MATLAB Function9/2(ym)
  Demux19/4 -> Scope43/4
  [I2] -> bdis13/1, bdis12/1, bdis11/1
  Unit Delay7/1 -> adis11/1, bdis15/1, Sum/1
  Mux17/1 -> Sum5/1, MATLAB Function12/1(ya)
  Signal Specification/1 -> MATLAB Function3/1(y_hat)
  bdis9/1 -> Sum/2
  MATLAB Function4/1(rol) -> Scope8/1
  MATLAB Function5/1(rol) -> Scope21/1
  Mux18/1 -> Sum11/1, MATLAB Function13/1(ya)
  Clock/1 -> MATLAB Function1/2(t)
  MATLAB Function6/1(rol) -> Scope16/1
  MATLAB Function3/2(norm_rd) -> To Workspace1/1, Scope39/1
  MATLAB Function5/3(m) -> Scope26/1
  bdis13/1 -> Sum24/2
  Delay2/1 -> MATLAB Function7/2(r1)
  Constant9/1 -> Mean (Variable Frequency)/1
  [I2] -> Mux10/2
  [I1] -> bdis14/1, bdis9/1, bdis8/1
  Mux15/1 -> Sum1/1, MATLAB Function8/1(ya)
  Demux5/4 -> Out3/1
  Demux3/3 -> Transfer Fcn3/1
  Unit Delay10/1 -> bdis16/1, adis12/1, Sum15/1
  MATLAB Function9/1(ruo2) -> Goto28/1, Scope48/1
  Sum/1 -> Demux4/1, Goto21/1, Scope47/1
  Demux5/2 -> Mux16/2
  Hw4/1 -> Mux13/1
  MATLAB Function7/2(Th_det) -> Mux14/2
  [u_fs] -> bdis7/1
  [V_vsi] -> Mux12/2
  [u_fs] -> bdis10/1
  Sum3/1 -> Demux6/1, Goto30/1, Scope49/1
  From57/1 -> MATLAB Function11/3(ruo2)
  Transfer Fcn1/1 -> Hw4/1
  bdis12/1 -> Sum15/2
  Sum14/1 -> Unit Delay7/1
  adis12/1 -> Sum16/3
  Signal Specification3/1 -> MATLAB Function11/2(x_hat2)
  bdis11/1 -> Sum16/2
  MATLAB Function13/1(ruo4) -> Goto36/1, Scope60/1
  Demux4/2 -> Mux15/2
  Sum24/1 -> Scope53/1
  Mean (Variable Frequency)1/1 -> Scope20/1
  MATLAB Function11/1(v2) -> Scope57/1
  From54/1 -> Signal Specification2/1
  [V_vsi] -> bdis20/1, bdis19/1, bdis18/1
  From50/1 -> Signal Specification5/1
  Signal Specification2/1 -> MATLAB Function11/1(x_hat1)
  bdis14/1 -> Sum23/2
  bdis16/1 -> Sum24/1
  Sum23/1 -> Scope52/1
  bdis15/1 -> Sum23/1
  Delay/1 -> MATLAB Function4/2(r1)
  bdis17/1 -> Sum9/1
  [I3] -> bdis4/1, bdis3/1, bdis2/1
  bdis19/1 -> Sum7/2
  cdis4/1 -> MATLAB Function1/1(y_hat), Scope35/1
  Sum6/1 -> Scope55/1
  bdis7/1 -> Sum14/1
  Demux3/2 -> Transfer Fcn2/1
  MATLAB Function5/2(xp) -> Integrator/1
  Demux4/3 -> Mux15/3
  Mux16/1 -> Sum2/1, MATLAB Function9/1(ya)
  Median Filter1/1 -> Scope18/1
  Transfer Fcn4/1 -> Hw3/1
  Demux4/1 -> Mux15/1
  [u_fs] -> bdis1/1
  MATLAB Function7/1(rol) -> Mux14/1
  Demux4/5 -> Mux15/4
  Sum1/1 -> Scope45/1
  Mean (Variable Frequency)/1 -> Scope19/1
  Demux5/1 -> Mux16/1
  bdis10/1 -> Sum16/1
  Unit Delay1/1 -> bdis6/1, adis1/1, Sum3/1
  MATLAB Function12/1(ruo3) -> Goto31/1, Scope51/1
  Sum8/1 -> Unit Delay6/1
  Sum7/1 -> Demux7/1, Goto32/1, Scope58/1
  Clock1/1 -> MATLAB Function3/3(tiempo)
  Sum5/1 -> Scope50/1
  Sum16/1 -> Unit Delay10/1
  Demux6/5 -> Mux17/4
  Signal Specification5/1 -> MATLAB Function10/1(x_hat1)
  Demux6/2 -> Mux17/2
  [I3] -> Mux11/2
  Hw2/1 -> Mux13/3
  Mux14/1 -> Scope42/1
  MATLAB Function2/1(y) -> Demux19/1
  adis11/1 -> Sum14/3
  MATLAB Function10/1(v1) -> Scope56/1
  bdis1/1 -> Sum4/1
  From56/1 -> MATLAB Function11/4(rol)
  Demux5/3 -> Mux16/3
  adis7/1 -> Sum8/3
  Demux7/5 -> Mux18/4
  Sum11/1 -> Scope59/1
  bdis2/1 -> Sum4/2
  Demux7/3 -> Mux18/3
  Demux7/1 -> Mux18/1
  bdis4/1 -> Sum6/2
  Signal Specification4/1 -> MATLAB Function10/2(x_hat2)
  [y_ma] -> Sum5/2, MATLAB Function12/2(ym)
  From53/1 -> MATLAB Function10/3(ruo1)
  adis1/1 -> Sum4/3
  Demux6/1 -> Mux17/1
  Unit Delay2/1 -> bdis21/1, adis2/1, Sum7/1
  Sum9/1 -> Unit Delay2/1
  From51/1 -> Signal Specification4/1
  From52/1 -> MATLAB Function10/4(rol)
  bdis20/1 -> Sum12/2
  bdis6/1 -> Sum6/1
  bdis18/1 -> Sum9/2
  bdis21/1 -> Sum12/1
  From55/1 -> Signal Specification3/1
  Sum2/1 -> Scope46/1
  Hw1/1 -> Mux13/2
  adis2/1 -> Sum9/3
  Demux4/4 -> Out2/1
  Demux6/4 -> Out4/1
  Mux13/1 -> Out1/1
  In1/1 -> Demux3/1
  Demux7/4 -> Out5/1

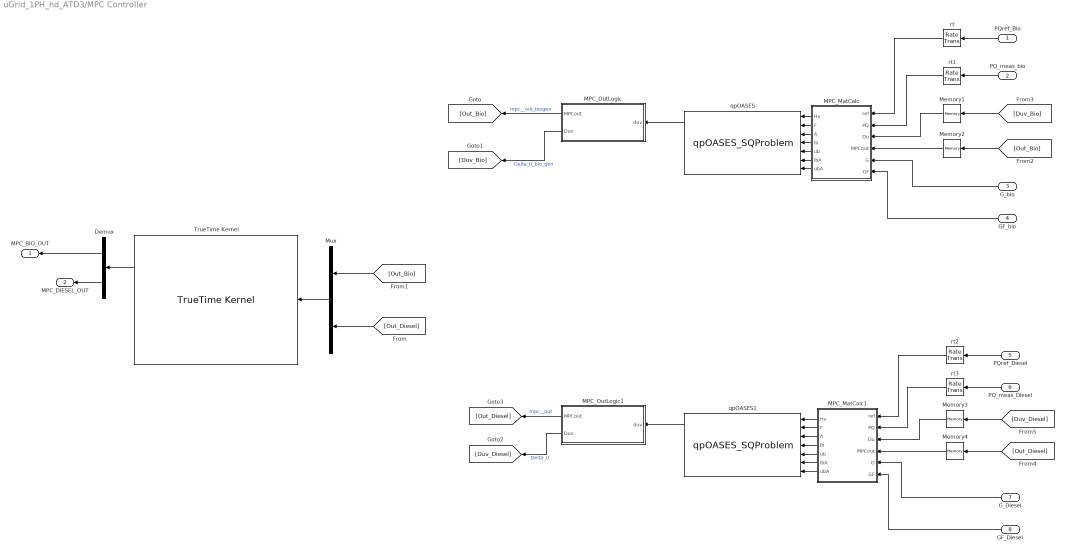
== system uGrid_1PH_hd_ATD3/MPC Controller ==
  PQref_Bio : Inport
  PQ_meas_bio : Inport  Port=2
  G_bio : Inport  Port=3
  GF_bio : Inport  Port=4
  PQref_Diesel : Inport  Port=5
  PQ_meas_Diesel : Inport  Port=6
  G_Diesel : Inport  Port=7
  GF_Diesel : Inport  Port=8
  Demux : Demux  Outputs=2
  MPC_MatCalc : MATLAB Function  TreatAsAtomicUnit=on  SystemSampleTime=1e-3
      settings: MinAlgLoopOccurrences=on
  MPC_MatCalc1 : MATLAB Function  TreatAsAtomicUnit=on  SystemSampleTime=1e-3
      settings: MinAlgLoopOccurrences=on
  MPC_OutLogic : MATLAB Function  TreatAsAtomicUnit=on
      settings: MinAlgLoopOccurrences=on
  MPC_OutLogic1 : MATLAB Function  TreatAsAtomicUnit=on
      settings: MinAlgLoopOccurrences=on
  Memory{1..4} (4 alike) : Memory
  Mux : Mux  Inputs=2
  TrueTime Kernel : truetime/TrueTime Kernel  sfun=MPC_PQ_init  args=[]  ninputsoutputs=[4 4]  ntriggers=0  trigtype=falling  nwnodenbr=[]  clockoffsetdrift=[0 0]  schedoutput=on  battery=off  poweroutput=off
  qpOASES : S-Function  FunctionName=qpOASES_SQProblem  SFunctionDeploymentMode=off  EnableBusSupport=off
  qpOASES1 : S-Function  FunctionName=qpOASES_SQProblem  SFunctionDeploymentMode=off  EnableBusSupport=off
  rt{,1..3} (4 alike) : RateTransition  InitialCondition=[0 0]  OutPortSampleTime=1e-3
  MPC_BIO_OUT : Outport
  MPC_DIESEL_OUT : Outport  Port=2
  wires:
  MPC_MatCalc/7(ubA) -> qpOASES/7
  G_bio/1 -> MPC_MatCalc/5(G)
  MPC_MatCalc/4(lb) -> qpOASES/4
  MPC_MatCalc/6(lbA) -> qpOASES/6
  Memory1/1 -> MPC_MatCalc/3(Du)
  rt1/1 -> MPC_MatCalc/2(PQ)
  GF_bio/1 -> MPC_MatCalc/6(GF)
  PQ_meas_bio/1 -> rt1/1
  MPC_MatCalc/2(F) -> qpOASES/2
  Memory2/1 -> MPC_MatCalc/4(MPCout)
  MPC_MatCalc/5(ub) -> qpOASES/5
  MPC_MatCalc/3(A) -> qpOASES/3
  rt/1 -> MPC_MatCalc/1(ref)
  MPC_MatCalc/1(Hv) -> qpOASES/1
  PQref_Bio/1 -> rt/1
  MPC_MatCalc1/7(ubA) -> qpOASES1/7
  G_Diesel/1 -> MPC_MatCalc1/5(G)
  MPC_MatCalc1/4(lb) -> qpOASES1/4
  MPC_MatCalc1/6(lbA) -> qpOASES1/6
  Memory3/1 -> MPC_MatCalc1/3(Du)
  rt3/1 -> MPC_MatCalc1/2(PQ)
  GF_Diesel/1 -> MPC_MatCalc1/6(GF)
  PQ_meas_Diesel/1 -> rt3/1
  MPC_MatCalc1/2(F) -> qpOASES1/2
  Memory4/1 -> MPC_MatCalc1/4(MPCout)
  MPC_MatCalc1/5(ub) -> qpOASES1/5
  MPC_MatCalc1/3(A) -> qpOASES1/3
  rt2/1 -> MPC_MatCalc1/1(ref)
  MPC_MatCalc1/1(Hv) -> qpOASES1/1
  PQref_Diesel/1 -> rt2/1
  [Duv_Bio] -> Memory1/1
  [Out_Bio] -> Memory2/1
  [Duv_Diesel] -> Memory3/1
  [Out_Diesel] -> Memory4/1
  qpOASES1/1 -> MPC_OutLogic1/1(duv)
  qpOASES/1 -> MPC_OutLogic/1(duv)
  MPC_OutLogic1/2(Duv) -> [Duv_Diesel]  "Delta_U"
  MPC_OutLogic/1(MPCout) -> [Out_Bio]  "mpc__out_biogen"
  MPC_OutLogic1/1(MPCout) -> [Out_Diesel]  "mpc__out"
  Mux/1 -> TrueTime Kernel/1
  MPC_OutLogic/2(Duv) -> [Duv_Bio]  "Delta_U_bio_gen"
  TrueTime Kernel/1 -> Demux/1
  Demux/2 -> MPC_DIESEL_OUT/1
  Demux/1 -> MPC_BIO_OUT/1
  [Out_Diesel] -> Mux/2
  [Out_Bio] -> Mux/1

== system uGrid_1PH_hd_ATD3/MeasureNode_I1 ==
  in : Inport
  Clock : Clock
  MATLAB Function : MATLAB Function  TreatAsAtomicUnit=on
  Pulse Generator1 : DiscretePulseGenerator  PulseType=Time based  Period=1e-4  PulseWidth=50  PhaseDelay=2e-3
  TrueTime Receive : truetime/TrueTime Receive  nwnbr=1  receiver=4  outdim=1  triggeroutput=on  senderoutput=off  lengthoutput=off  priorityoutput=off  timestampoutput=off  signalpoweroutput=off  msgIDoutput=off
  TrueTime Send : truetime/TrueTime Send  trigger=falling  nwnbr=1  sender=3  indim=1  recsource=internal  receiver=4  lengthsource=internal  length=10000  priosource=internal  prio=1  msgIDsource=internal  msgID=0  dynamicSegment=dynamic
  Out : Outport
  wires:
  Pulse Generator1/1 -> TrueTime Send/2
  TrueTime Receive/1 -> Out/1
  Clock/1 -> MATLAB Function/1(u1)
  MATLAB Function/1(y) -> TrueTime Send/1
  in/1 -> MATLAB Function/2(u2)

== system uGrid_1PH_hd_ATD3/MeasureNode_I2 ==
  in : Inport
  Clock : Clock
  MATLAB Function : MATLAB Function  TreatAsAtomicUnit=on
  Pulse Generator1 : DiscretePulseGenerator  PulseType=Time based  Period=1e-4  PulseWidth=50  PhaseDelay=1e-3
  TrueTime Receive : truetime/TrueTime Receive  nwnbr=1  receiver=2  outdim=1  triggeroutput=on  senderoutput=off  lengthoutput=off  priorityoutput=off  timestampoutput=off  signalpoweroutput=off  msgIDoutput=off
  TrueTime Send : truetime/TrueTime Send  trigger=falling  nwnbr=1  sender=1  indim=1  recsource=internal  receiver=2  lengthsource=internal  length=10000  priosource=internal  prio=1  msgIDsource=internal  msgID=0  dynamicSegment=dynamic
  Out : Outport
  wires:
  TrueTime Receive/1 -> Out/1
  Pulse Generator1/1 -> TrueTime Send/2
  Clock/1 -> MATLAB Function/1(u1)
  MATLAB Function/1(y) -> TrueTime Send/1
  in/1 -> MATLAB Function/2(u2)

== system uGrid_1PH_hd_ATD3/MeasureNode_I3 ==
  in : Inport
  Clock : Clock
  MATLAB Function : MATLAB Function  TreatAsAtomicUnit=on
  Pulse Generator1 : DiscretePulseGenerator  PulseType=Time based  Period=1e-4  PulseWidth=50  PhaseDelay=3e-3
  TrueTime Receive : truetime/TrueTime Receive  nwnbr=1  receiver=6  outdim=1  triggeroutput=on  senderoutput=off  lengthoutput=off  priorityoutput=off  timestampoutput=off  signalpoweroutput=off  msgIDoutput=off
  TrueTime Send : truetime/TrueTime Send  trigger=falling  nwnbr=1  sender=5  indim=1  recsource=internal  receiver=6  lengthsource=internal  length=10000  priosource=internal  prio=1  msgIDsource=internal  msgID=0  dynamicSegment=dynamic
  Out : Outport
  wires:
  in/1 -> MATLAB Function/2(u2)
  Pulse Generator1/1 -> TrueTime Send/2
  TrueTime Receive/1 -> Out/1
  Clock/1 -> MATLAB Function/1(u1)
  MATLAB Function/1(y) -> TrueTime Send/1

== system uGrid_1PH_hd_ATD3/MeasureNode_I4 ==
  in : Inport
  Clock : Clock
  MATLAB Function : MATLAB Function  TreatAsAtomicUnit=on
  Pulse Generator1 : DiscretePulseGenerator  PulseType=Time based  Period=1e-4  PulseWidth=50  PhaseDelay=4e-3
  TrueTime Receive : truetime/TrueTime Receive  nwnbr=1  receiver=8  outdim=1  triggeroutput=on  senderoutput=off  lengthoutput=off  priorityoutput=off  timestampoutput=off  signalpoweroutput=off  msgIDoutput=off
  TrueTime Send : truetime/TrueTime Send  trigger=falling  nwnbr=1  sender=7  indim=1  recsource=internal  receiver=8  lengthsource=internal  length=10000  priosource=internal  prio=1  msgIDsource=internal  msgID=0  dynamicSegment=dynamic
  Out : Outport
  wires:
  Pulse Generator1/1 -> TrueTime Send/2
  TrueTime Receive/1 -> Out/1
  in/1 -> MATLAB Function/2(u2)
  MATLAB Function/1(y) -> TrueTime Send/1
  Clock/1 -> MATLAB Function/1(u1)

== system uGrid_1PH_hd_ATD3/Subsystem ==
  Battery : electricdrivelib/Extra Sources/Battery  BatType=Lithium-Ion  ShowTempParam=off  ThermalPreset=no  ShowAgeParam=off  NomV=1000  NomQ=20  SOC=100  Batt_Tr=10e-3  PresetModel=off  MaxQ=1  MinV=825  FullV=1280.3859  Dis_rate=200  R=50e-3  Normal_OP=0.90435  expZone="[1188.4244    0.049130435]"  current=[6.5 13 32.5 50]  Units=Time  Tci=20  NomT=20  T2=-30  MaxQ2=4.8  FullV2=7.1  Normal_OP2=5.655  expZone2="[6.58           1]"  Rca=0.6  ti=2000  Dp=0  Neq0=0  Tsim=1e6  Ta1=25  Qeol=5.4*0.9  Reol=0.013333*1.2  Char_age=[2.3478, 3]  Dis_age=[2.3478, 10]  N1=1500  N2=10500  N3=1000  N4=1400  Ta2=45  N5=950
  Constant2 : Constant  Value=1000
  Constant4 : Constant  Value=25
  Controlled Current Source : powerlib/Electrical Sources/Controlled Current Source  Initialize=on  Source_Type=AC  Amplitude=0  Phase=0  Frequency=0  Measurements=None
  Gain3 : Gain  Gain=1/10
  PV panel1 : Subsystem
      mask Display: image('panel.jpg')
  Rcable : powerlib/Elements/Series RLC Branch  LConnTagsString=__new0  RConnTagsString=__new0  BranchType=R  Resistance=1e-3  Inductance=1e-3  SetiL0=off  InitialCurrent=0  Capacitance=1e-6  Setx0=off  InitialVoltage=0  Measurements=None
  Rin2 : powerlib/Elements/Series RLC Branch  LConnTagsString=__new0  RConnTagsString=__new0  BranchType=C  Resistance=.001  Inductance=0  SetiL0=off  InitialCurrent=0  Capacitance=1000e-6  Setx0=off  InitialVoltage=0  Measurements=None
  + : PMIOPort  Side=Left
  - : PMIOPort  Port=2  Side=Left
  Out1 : Outport
  wires:
  PV panel1/1(I) -> Gain3/1
  Gain3/1 -> Controlled Current Source/1
  Battery/1 -> Out1/1
  Constant4/1 -> PV panel1/3(Top)
  Constant2/1 -> PV panel1/2(G)
  [V] -> PV panel1/1(V)
  connections:
  Rcable/RConn1 -- +/RConn1
  Battery/LConn1 -- Controlled Current Source/RConn1 -- Rcable/LConn1 -- Rin2/LConn1
  Battery/LConn2 -- -/RConn1 -- Rin2/RConn1 -- Controlled Current Source/LConn1

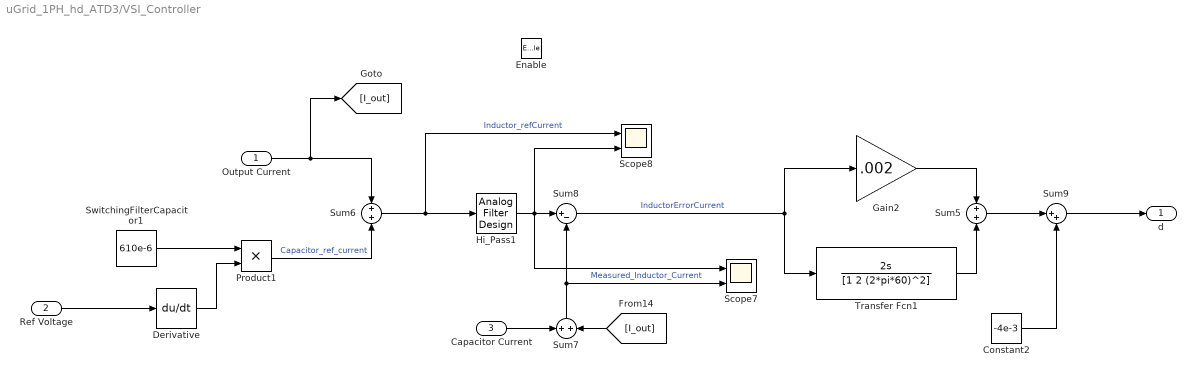
== system uGrid_1PH_hd_ATD3/VSI_Controller ==
  Output Current : Inport
  Ref Voltage : Inport  Port=2
  Capacitor Current : Inport  Port=3
  Enable : EnablePort
  Constant2 : Constant  Value=-4e-3
  Derivative : Derivative  CoefficientInTFapproximation=1e-3
  Gain2 : Gain  Gain=.002
  Hi_Pass1 : dsparch4/Analog Filter Design  method=Bessel  filttype=Highpass  N=1  Wlo=1*2*pi  Whi=80  Rp=2  Rs=40
  Product1 : Product
  Scope7 : Scope  NumInputPorts=2
  Scope8 : Scope  NumInputPorts=2
  Sum5 : Sum  Inputs=+|+
  Sum6 : Sum  Inputs=+|+
  Sum7 : Sum  Inputs=+|+
  Sum8 : Sum  Inputs=|+-
  Sum9 : Sum  Inputs=|++
  SwitchingFilterCapacitor1 : Constant  Value=610e-6
  Transfer Fcn1 : TransferFcn  Numerator=[2 0]  Denominator=[1 2 (2*pi*60)^2]
  d : Outport
  wires:
  Derivative/1 -> Product1/2
  Sum6/1 -> Hi_Pass1/1, Scope8/1  "Inductor_refCurrent"
  Sum8/1 -> Transfer Fcn1/1, Gain2/1  "InductorErrorCurrent"
  Ref Voltage/1 -> Derivative/1
  Constant2/1 -> Sum9/2
  Capacitor Current/1 -> Sum7/1
  Transfer Fcn1/1 -> Sum5/2
  Output Current/1 -> Sum6/1, [I_out]
  [I_out] -> Sum7/2
  Gain2/1 -> Sum5/1
  SwitchingFilterCapacitor1/1 -> Product1/1
  Hi_Pass1/1 -> Scope8/2, Sum8/1, Scope7/1
  Product1/1 -> Sum6/2  "Capacitor_ref_current"
  Sum9/1 -> d/1
  Sum5/1 -> Sum9/1
  Sum7/1 -> Scope7/2, Sum8/2  "Measured_Inductor_Current"

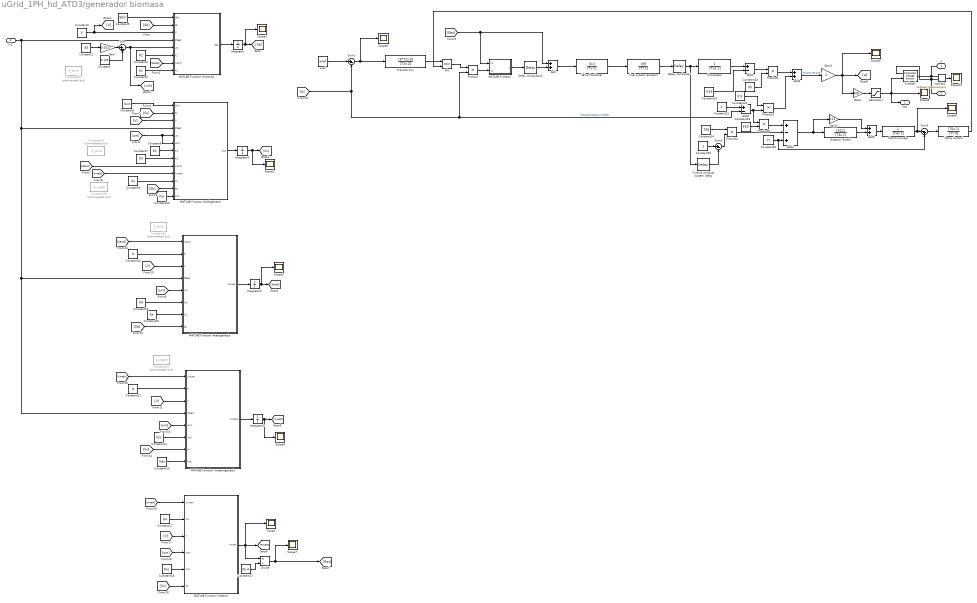
== system uGrid_1PH_hd_ATD3/generador biomasa ==
  In1 : Inport
  Add : Sum
  Add1 : Sum  Inputs=+-
  Add2 : Sum
  Add3 : Sum  Inputs=+-
  Add4 : Sum  Inputs=+-+
  Add5 : Sum
  Compresor : TransferFcn  Denominator=[Tcd 1]
  Constant : Constant  Value=0.129
  Constant1 : Constant  Value=35
  Constant10 : Constant  Value=Ksc
  Constant11 : Constant  Value=b
  Constant12 : Constant  Value=b
  Constant13 : Constant  Value=Kdc
  Constant14 : Constant  Value=Ksc
  Constant15 : Constant  Value=Ks
  Constant16 : Constant  Value=Kd
  Constant17 : Constant  Value=K4
  Constant18 : Constant  Value=Ksc
  Constant19 : Constant  Value=K33
  Constant2 : Constant  Value=Ks
  Constant20 : Constant  Value=Kh
  Constant21 : Constant
  Constant22 : Constant  Value=0.5
  Constant23 : Constant  Value=550
  Constant24 : Constant  Value=700
  Constant25 : Constant
  Constant26 : Constant  Value=Tr
  Constant27 : Constant  Value=35.4
  Constant28 : Constant  Commented=on  Value=X_acid
  Constant29 : Constant  Commented=on  Value=X_acid
  Constant3 : Constant  Value=V
  Constant30 : Constant  Commented=on  Value=X_meth
  Constant31 : Constant  Commented=on  Value=X_acid
  Constant32 : Constant  Commented=on  Value=X_meth
  Constant4 : Constant  Value=K1
  Constant5 : Constant  Value=Sbin
  Constant6 : Constant  Value=Svin
  Constant7 : Constant  Value=K3
  Constant8 : Constant  Value=K2
  Constant9 : Constant  Value=Ks
  Delay combustor : TransportDelay  DelayTime=Tcr
  Delay combustor1 : TransportDelay  DelayTime=0
  Divide : Product  Inputs=*/
  Fuel system actuator : TransferFcn  Numerator=[Kf]  Denominator=[Tf C]
  Gain : Gain  Gain=0.013
  Gain1 : Gain  Gain=900
  Gain2 : Gain  Gain=K11
  Gain3 : Gain
  Integrator : Integrator
  Integrator1 : Integrator
  Integrator2 : Integrator  InitialCondition=1.2
  Integrator3 : Integrator  InitialCondition=0.35
  MATLAB Function : MATLAB Function  TreatAsAtomicUnit=on
  MATLAB Function Acetogenesis : MATLAB Function  TreatAsAtomicUnit=on
  MATLAB Function Acidogenesis : MATLAB Function  TreatAsAtomicUnit=on
  MATLAB Function Hidrolisis : MATLAB Function  TreatAsAtomicUnit=on
  MATLAB Function metano : MATLAB Function  TreatAsAtomicUnit=on
  MATLAB Function metanogenesis : MATLAB Function  TreatAsAtomicUnit=on
  Min : MinMax  Inputs=2
  Product{,1..4} (5 alike) : Product
  Rotation Shield : TransferFcn  Numerator=[K22]  Denominator=[T3s 1]
  Saturation : Saturate  UpperLimit=1000  LowerLimit=0
  Scope{,1..10} (11 alike) : Scope
  Sum : Sum  Inputs=|+-
  Sum1 : Sum  Inputs=|+-
  Sum2 : Sum  Inputs=|+-
  Sum3 : Sum  Inputs=|-+
  Temp Control : TransferFcn  Numerator=[T5s 1]  Denominator=[Tt 0]
  Transfer Fcn : TransferFcn  Numerator=[K*T1s K]  Denominator=[T2s Z]
  Turbine exhaust system delay : TransportDelay  DelayTime=Ttd
  V_diesel : powerlib/Electrical Sources/Controlled Voltage Source  Initialize=on  Source_Type=DC  Amplitude=0  Phase=0  Frequency=0  Measurements=None
  Valve Positioner : TransferFcn  Numerator=[Kv]  Denominator=[Tv C]
  Vsensa1 : powerlib/Measurements/Voltage Measurement  PhasorSimulation=off  OutputType=Complex  PSBequivalent=0
  thermo couple : TransferFcn  Denominator=[T4s 1]
  wref : Constant  Value=wref
  + : PMIOPort  Side=Left
  - : PMIOPort  Port=2  Side=Left
  Vdc : Outport
  wires:
  MATLAB Function metano/1(Fmeth) -> Divide/1, Scope/1, [Fmeth]
  Sum/1 -> [um], MATLAB Function Hidrolisis/5(um)
  Constant16/1 -> MATLAB Function Acetogenesis/6(Kd)
  Temp Control/1 -> Min/2
  Integrator/1 -> Scope1/1, [Sb]
  Gain3/1 -> Gain1/1, Scope5/1, [w]
  Sum1/1 -> Transfer Fcn/1, Scope6/1
  [Sb] -> MATLAB Function Acetogenesis/8(Sb)
  [Sv] -> MATLAB Function metanogenesis/7(Sv)
  Add4/1 -> Rotation Shield/1, Gain2/1
  Constant8/1 -> MATLAB Function Acidogenesis/7(K2)
  Constant24/1 -> Product4/1
  [V] -> MATLAB Function Acetogenesis/3(V)
  Constant23/1 -> Product3/2
  Constant27/1 -> Divide/2
  [Sb] -> MATLAB Function Acidogenesis/12(Sb)
  Integrator3/1 -> Scope4/1, [Xmeth]
  Integrator2/1 -> Scope3/1, [Xacid]
  Divide/1 -> Scope7/1, [Gas]
  Constant7/1 -> MATLAB Function Acidogenesis/8(K3)
  Delay combustor/1 -> Turbine exhaust system delay/1, Compresor/1
  [V] -> MATLAB Function Acidogenesis/3(V)
  Constant12/1 -> MATLAB Function Acetogenesis/2(b)
  Sum2/1 -> Product4/2
  [V] -> MATLAB Function metanogenesis/3(V)
  Gain/1 -> Sum/1
  Product/1 -> MATLAB Function/2(u2)
  [w] -> Product/2, Add3/2, Sum1/2  "velocidad angular medida"
  Constant6/1 -> MATLAB Function Acidogenesis/1(Svin)
  wref/1 -> Sum1/1
  [Gas] -> MATLAB Function/1(u1), Add/1
  [Sv] -> MATLAB Function metano/6(Sv)
  MATLAB Function Hidrolisis/1(Sbp) -> Integrator/1
  Turbine exhaust system delay/1 -> Sum2/2
  MATLAB Function Acetogenesis/1(Xacidp) -> Integrator2/1
  Constant/1 -> Sum/2
  Constant18/1 -> MATLAB Function metano/5(Ksc)
  In1/1 -> MATLAB Function Acidogenesis/4(Ffeed), MATLAB Function metanogenesis/4(Ffeed), MATLAB Function Acetogenesis/4(Ffeed), MATLAB Function Hidrolisis/4(Ffeed)
  Add3/1 -> Product3/1, Product2/2
  [um] -> MATLAB Function Acetogenesis/5(um)
  Product3/1 -> Add4/1
  Constant15/1 -> MATLAB Function Acetogenesis/7(Ks)
  thermo couple/1 -> Scope8/1, Sum3/1
  Fuel system actuator/1 -> Delay combustor/1
  Add/1 -> Valve Positioner/1
  Add5/1 -> thermo couple/1
  Gain2/1 -> Add5/1
  Constant22/1 -> Product2/1
  [um] -> MATLAB Function metano/4(umc)
  Compresor/1 -> Add1/1
  Constant10/1 -> MATLAB Function Acidogenesis/13(Ksc)
  [um] -> MATLAB Function Acidogenesis/6(umc), MATLAB Function Acidogenesis/5(um)
  Constant9/1 -> MATLAB Function Acidogenesis/11(Ks)
  Constant1/1 -> Gain/1
  Constant13/1 -> MATLAB Function metanogenesis/8(Kdc)
  Constant26/1 -> Sum3/2, Add4/3
  Integrator1/1 -> Scope2/1, [Sv]
  [Xmeth] -> MATLAB Function metanogenesis/1(Xmeth)
  Add2/1 -> Gain3/1  "Torque mecánico"
  MATLAB Function/1(y) -> Delay combustor1/1
  Saturation/1 -> Vdc/1, V_diesel/1, Scope9/1
  [Sb] -> MATLAB Function Hidrolisis/2(Sb)
  Min/1 -> Product/1
  Constant3/1 -> [V], MATLAB Function Hidrolisis/3(V)
  MATLAB Function Acidogenesis/1(Svp) -> Integrator1/1
  Constant5/1 -> MATLAB Function Hidrolisis/1(Sbin)
  Constant20/1 -> Product1/2
  [Xmeth] -> MATLAB Function Acidogenesis/10(Xmeth)
  Sum3/1 -> Temp Control/1
  Gain1/1 -> Saturation/1
  Constant21/1 -> Add3/1
  Constant25/1 -> Sum2/1
  Product2/1 -> Add2/2
  [Xacid] -> MATLAB Function Acidogenesis/9(Xacid)
  Valve Positioner/1 -> Fuel system actuator/1
  Constant4/1 -> MATLAB Function Hidrolisis/6(K1)
  Constant11/1 -> MATLAB Function metanogenesis/2(b)
  Rotation Shield/1 -> Add5/2
  Add1/1 -> Product1/1
  [Sv] -> MATLAB Function Acidogenesis/2(Sv)
  [Xacid] -> MATLAB Function Acetogenesis/1(Xacid)
  Constant19/1 -> Add1/2
  Product1/1 -> Add2/1
  Transfer Fcn/1 -> Min/1
  Delay combustor1/1 -> Add/2
  [um] -> MATLAB Function metanogenesis/5(umc)
  MATLAB Function metanogenesis/1(Xmethp) -> Integrator3/1
  Constant14/1 -> MATLAB Function metanogenesis/6(Ksc)
  Product4/1 -> Add4/2
  Constant2/1 -> MATLAB Function Hidrolisis/8(Ks)
  Constant17/1 -> MATLAB Function metano/2(K4)
  [V] -> MATLAB Function metano/3(V)
  [Xmeth] -> MATLAB Function metano/1(Xmeth)
  [Xacid] -> MATLAB Function Hidrolisis/7(Xacid)
  Vsensa1/1 -> Scope10/1
  connections:
  V_diesel/RConn1 -- Vsensa1/LConn1 -- +/RConn1
  V_diesel/LConn1 -- Vsensa1/LConn2 -- -/RConn1
